simulink model "sldemo_mdlref_datamngt"  (Simulink 7.6)
settings: Solver=FixedStepDiscrete  SolverMode=SingleTasking  StartTime=0.0  StopTime=10.0  RelTol=1e-3
PreLoadFcn:
  | sldemo_mdlref_datamngt_wsdata
  | sldemo_mdlref_counter_datamngt_types
undefined symbols (not defined in the file or in its folder): CounterICs, CounterParams
libraries: sldemo_mdlref_counter_datamngt_lib x3
settings Model: Creator=The MathWorks Inc.  ExtModeAutoUpdateStatusClock=off
settings DataIOCC: SaveFormat=StructureWithTime  SaveOutput=off  SignalLogging=off  DSMLogging=off  SaveTime=off  SignalLoggingName=logsOut
settings OptimizationCC: InlineParams=on  InlineInvariantSignals=on  EnhancedBackFolding=on  StrengthReduction=on  StateBitsets=on  DataBitsets=on  UseTempVars=on  EfficientFloat2IntCast=on
settings DebuggingCC: SaveWithParameterizedLinksMsg=none  UnderspecifiedInitializationDetection=Simplified  CheckExecutionContextPreStartOutputMsg=on  CheckExecutionContextRuntimeOutputMsg=on  SolverPrmCheckMsg=none  MultiTaskDSMMsg=warning  MultiTaskCondExecSysMsg=none  SigSpecEnsureSampleTimeMsg=none  StrictBusMsg=ErrorOnBusTreatedAsVector
settings HardwareCC: TargetHWDeviceType=32-bit Generic
settings ModelReferenceCC: UpdateModelReferenceTargets=IfOutOfDate  CheckModelReferenceTargetMessage=none
settings RTWCC: GenerateReport=on  RTWVerbose=off  ProcessScript=grt_make_rtw_hook  LaunchReport=on  IncludeERTFirstTime=on
settings CodeAppCC: ForceParamTrailComments=on  MaxIdLength=100
settings GRTTargetCC: MatFileLogging=off

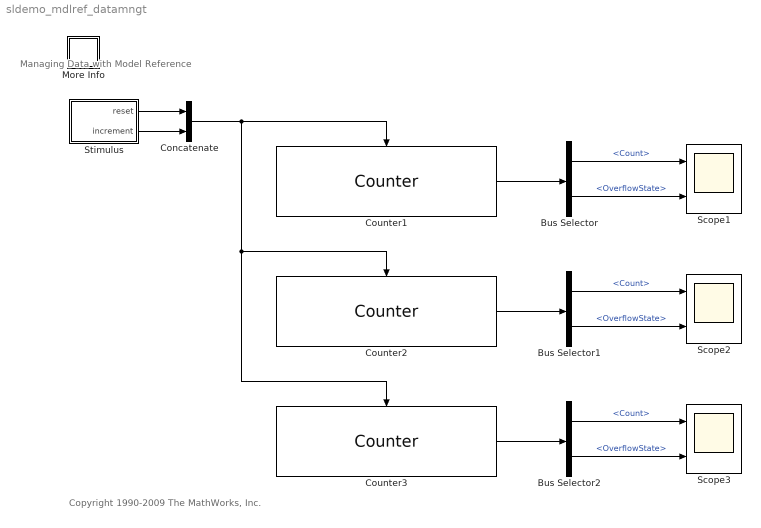
== system sldemo_mdlref_datamngt ==
  note: Managing Data with Model Reference
  note: Copyright 1990-2009 The MathWorks, Inc.
  Bus Selector : BusSelector  OutputSignals=Count,OverflowState
  Bus Selector1 : BusSelector  OutputSignals=Count,OverflowState
  Bus Selector2 : BusSelector  OutputSignals=Count,OverflowState
  Concatenate : Concatenate  Mode=Vector
  Counter1 : sldemo_mdlref_counter_datamngt_lib/Counter  ParameterArgumentNames=CounterParams,CounterICs  ParameterArgumentValues=Params, ICs  SimulationMode=Normal  ModelReferenceVersion=1.2  DefaultDataLogging=off  TriggerPortName=Trigger on rising edge  TriggerPortTriggerType=rising  Params=Param1  ICs=IC1
  Counter2 : sldemo_mdlref_counter_datamngt_lib/Counter  ParameterArgumentNames=CounterParams,CounterICs  ParameterArgumentValues=Params, ICs  SimulationMode=Accelerator  ModelReferenceVersion=1.2  DefaultDataLogging=off  TriggerPortName=Trigger on rising edge  TriggerPortTriggerType=rising  Params=Param2  ICs=IC1
  Counter3 : sldemo_mdlref_counter_datamngt_lib/Counter  ParameterArgumentNames=CounterParams,CounterICs  ParameterArgumentValues=Params, ICs  SimulationMode=Accelerator  ModelReferenceVersion=1.2  DefaultDataLogging=off  TriggerPortName=Trigger on rising edge  TriggerPortTriggerType=rising  Params=Param2  ICs=IC2
  More Info : Subsystem
      settings: OpenFcn=showdemo(bdroot(gcb))
      mask Display: disp('?')
  Scope1 : Scope  NumInputPorts=2
      settings: TimeRange=10  YMin=-21~-2  YMax=21~2
  Scope2 : Scope  NumInputPorts=2
      settings: TimeRange=10  YMin=-21~-2  YMax=21~2  SaveName=ScopeData2
  Scope3 : Scope  NumInputPorts=2
      settings: TimeRange=10  YMin=-21~-2  YMax=21~2  SaveName=ScopeData3
  Stimulus : Subsystem  mask(Counter Input Stimulus){ResetPeriod=4, IncrementPeriod=0.2, SampleTime=0.1}
      mask prompts: ResetPeriod "Period for resetting counter:"; IncrementPeriod "Period for incrementing counter:"; SampleTime "Sample time:"
      mask help:
      | Provide input signals for driving counters.  Parameters control:
      | - The frequency of the input pulses to be counted.
      | - The frequency with which the counter should be reset.
  wires:
  Counter1/1 -> Bus Selector/1
  Bus Selector/1 -> Scope1/1  "<Count>"
  Bus Selector/2 -> Scope1/2  "<OverflowState>"
  Concatenate/1 -> Counter2/Trigger, Counter3/Trigger, Counter1/Trigger
  Counter2/1 -> Bus Selector1/1
  Bus Selector1/1 -> Scope2/1  "<Count>"
  Bus Selector1/2 -> Scope2/2  "<OverflowState>"
  Counter3/1 -> Bus Selector2/1
  Bus Selector2/1 -> Scope3/1  "<Count>"
  Bus Selector2/2 -> Scope3/2  "<OverflowState>"
  Stimulus/1(reset) -> Concatenate/1
  Stimulus/2(increment) -> Concatenate/2

== system sldemo_mdlref_datamngt/More Info ==
  note: This demonstration uses model arguments defined as parameter structures
      | to parameterize three instances of a referenced model that implements a
      | triggered counter algorithm.
  note: Bus Block Demonstration

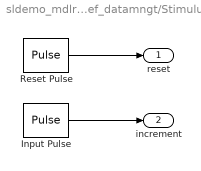
== system sldemo_mdlref_datamngt/Stimulus ==
  Input Pulse : DiscretePulseGenerator  Amplitude=logical(1)  Period=round(IncrementPeriod/SampleTime)  SampleTime=SampleTime  VectorParams1D=off
  Reset Pulse : DiscretePulseGenerator  Amplitude=logical(1)  Period=round(ResetPeriod/SampleTime)  SampleTime=SampleTime  VectorParams1D=off
  reset : Outport
  increment : Outport  Port=2
  wires:
  Input Pulse/1 -> increment/1
  Reset Pulse/1 -> reset/1
